simulink model "top12x17"  (Simulink 6.3)
settings: Solver=FixedStepDiscrete  StartTime=0.0  StopTime=5000  FixedStep=1  RelTol=1e-3
PreLoadFcn:
  | FifoDepth=17;
  | SymbolWidth = 8;
InitFcn:
  | %% DSPBuilder Start
  | alt_dspbuilder_update_model(bdroot)
  | %% DSPBuilder End
libraries: allblocks_alteradspbuilder2 x98, simulink x1
settings Model: LastModifiedBy=LKONG  StrictBusMsg=None
settings DataIOCC: SignalLoggingName=sigsOut
settings OptimizationCC: BooleanDataType=off  InlineInvariantSignals=on
settings DebuggingCC: SolverPrmCheckMsg=none
settings HardwareCC: TargetUnknown=on

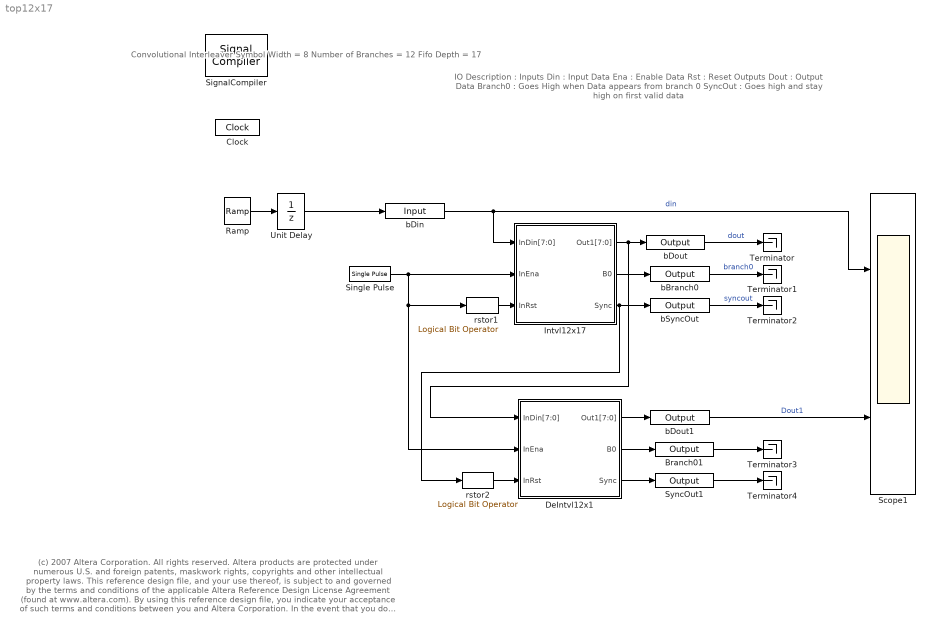
== system top12x17 ==
  note: (c) 2007 Altera Corporation. All rights reserved.  Altera products are protected under numerous U.S. and foreign patents, maskwork rights, copyrights and other intellectual property laws.
      | This reference design file, and your use thereof, is subject to and governed by the terms and conditions of the applicable Altera Reference Design License Agreement (found at www.altera.com).
      | By using this reference design file, you indicate your acceptance of such terms and conditions between you and Altera Corporation.
      | In the event that you do not agree with such terms and conditions, you may not use the reference design file and please promptly destroy any copies you have made.
      | This reference design file being provided on an "as-is" basis and as an accommodation and therefore all warranties, representations or guarantees of any kind (whether express, implied or statutory)
      | including, without limitation, warranties of merchantability, non-infringement, or fitness for a particular purpose, are specifically disclaimed.
      | By making this reference design file available, Altera expressly does not recommend, suggest or require that this reference design file be used in combination with any other product not provided by Altera
  note: IO Description :
      |
      | Inputs
      |            Din    : Input Data
      |            Ena   : Enable Data
      |            Rst    : Reset
      |
      | Outputs
      |           Dout        : Output Data
      |           Branch0 : Goes High when Data appears from branch 0
      |           SyncOut : Goes high and stay high on first valid data
  note: Convolutional Interleaver
      | Symbol Width = 8
      | Number of Branches = 12
      | Fifo Depth = 17
  Branch01 : allblocks_alteradspbuilder2/Output  iofile=d:\wsTrunk\workspace\Documentation\DesignExamples\Demos\Transforms\CrossInterleaver12x17\tb_top12x17\top12x17_Branch01.capture  BusType=Single Bit  bwl=1  bwr=0  PORTTYPE=Output
  Clock : allblocks_alteradspbuilder2/Clock  ClockPeriod=100  ClockPeriodUnit=ns  SampleTime=1  SimulationStartCycle=5  PhaseOffset=0  Reset=aclr  ResetType=Active Low  Export=off
  DeIntvl12x1 : Subsystem  AncestorBlock=ALTELINK/AltLab/HDL SubSystem
      mask Type: SubSystem AlteraBlockSet
  Intvl12x17 : Subsystem  AncestorBlock=ALTELINK/AltLab/HDL SubSystem
      mask Type: SubSystem AlteraBlockSet
  Ramp : simulink/Sources/Ramp  slope=1  start=0  X0=3
  Scope1 : Scope  NumInputPorts=2
      settings: TimeRange=3000  YMin=-5~-150  YMax=5~150
  SignalCompiler : allblocks_alteradspbuilder2/Signal Compiler  DeviceFamily=Cyclone IV GX  DeviceName=AUTO  EnableSignalTap=off  SignalTapDepth=128  UseBoardBlock=off  StpUseDefaultClock=on  StpClock=Clock
  Single Pulse : allblocks_alteradspbuilder2/Single Pulse  signal_type=Step Up  impulse_width=1  delay=1  SpecifyClock=off  use_ena=off  use_sclr=off
  SyncOut1 : allblocks_alteradspbuilder2/Output  iofile=d:\wsTrunk\workspace\Documentation\DesignExamples\Demos\Transforms\CrossInterleaver12x17\tb_top12x17\top12x17_SyncOut1.capture  BusType=Single Bit  bwl=1  bwr=0  PORTTYPE=Output
  Terminator{,1..4} (5 alike) : Terminator
  Unit Delay : UnitDelay
  bBranch0 : allblocks_alteradspbuilder2/Output  iofile=d:\wsTrunk\workspace\Documentation\DesignExamples\Demos\Transforms\CrossInterleaver12x17\tb_top12x17\top12x17_bBranch0.capture  BusType=Single Bit  bwl=1  bwr=0  PORTTYPE=Output
  bDin : allblocks_alteradspbuilder2/Input  iofile=d:\wsTrunk\workspace\Documentation\DesignExamples\Demos\Transforms\CrossInterleaver12x17\tb_top12x17\top12x17_bDin.salt  BusType=Signed Integer  bwl=8  bwr=0  SpecifyClock=off  PORTTYPE=Input
  bDout : allblocks_alteradspbuilder2/Output  iofile=d:\wsTrunk\workspace\Documentation\DesignExamples\Demos\Transforms\CrossInterleaver12x17\tb_top12x17\top12x17_bDout.capture  BusType=Signed Integer  bwl=8  bwr=0  PORTTYPE=Output
  bDout1 : allblocks_alteradspbuilder2/Output  iofile=d:\wsTrunk\workspace\Documentation\DesignExamples\Demos\Transforms\CrossInterleaver12x17\tb_top12x17\top12x17_bDout1.capture  BusType=Signed Integer  bwl=8  bwr=0  PORTTYPE=Output
  bSyncOut : allblocks_alteradspbuilder2/Output  iofile=d:\wsTrunk\workspace\Documentation\DesignExamples\Demos\Transforms\CrossInterleaver12x17\tb_top12x17\top12x17_bSyncOut.capture  BusType=Single Bit  bwl=1  bwr=0  PORTTYPE=Output
  rstor1 : allblocks_alteradspbuilder2/Logical Bit Operator  LogicalOperator=NOT  user_inputs=2
  rstor2 : allblocks_alteradspbuilder2/Logical Bit Operator  LogicalOperator=NOT  user_inputs=2
  wires:
  Intvl12x17/1(Out1[7:0]) -> bDout/1, DeIntvl12x1/1(InDin[7:0])
  bDin/1 -> Scope1/1, Intvl12x17/1(InDin[7:0])  "din"
  Single Pulse/1 -> Intvl12x17/2(InEna), rstor1/1, DeIntvl12x1/2(InEna)
  rstor1/1 -> Intvl12x17/3(InRst)
  Ramp/1 -> Unit Delay/1
  Intvl12x17/2(B0) -> bBranch0/1
  Intvl12x17/3(Sync) -> bSyncOut/1, rstor2/1
  Unit Delay/1 -> bDin/1
  rstor2/1 -> DeIntvl12x1/3(InRst)
  DeIntvl12x1/1(Out1[7:0]) -> bDout1/1
  DeIntvl12x1/2(B0) -> Branch01/1
  DeIntvl12x1/3(Sync) -> SyncOut1/1
  bDout/1 -> Terminator/1  "dout"
  bBranch0/1 -> Terminator1/1  "branch0"
  bSyncOut/1 -> Terminator2/1  "syncout"
  Branch01/1 -> Terminator3/1
  SyncOut1/1 -> Terminator4/1
  bDout1/1 -> Scope1/2  "Dout1"

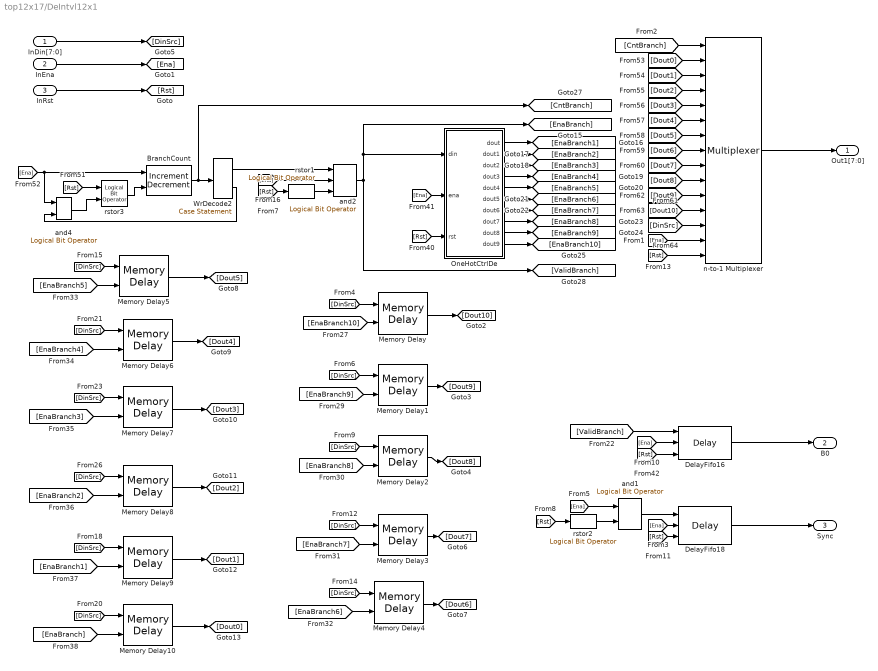
== system top12x17/DeIntvl12x1 ==
  InDin[7:0] : Inport
  InEna : Inport  Port=2
  InRst : Inport  Port=3
  BranchCount : allblocks_alteradspbuilder2/Increment Decrement  BusType=Unsigned Integer  bwl=4  bwr=0  SpecifyClock=off  clr_value=0  direction=Increment  phase_selection=1  use_ena=on  use_sclr=on
  DelayFifo16 : allblocks_alteradspbuilder2/Delay  pipeline=2  ClockPhase=1  use_ena=on  use_sclr=on  use_init=off  reset_value=1
  DelayFifo18 : allblocks_alteradspbuilder2/Delay  pipeline=2  ClockPhase=1  use_ena=on  use_sclr=on  use_init=off  reset_value=1
  Memory Delay : allblocks_alteradspbuilder2/Memory Delay  BusType=Inferred  bwl=8  bwr=0  pipeline=17  ram_type=AUTO  use_ena=on  use_sclr=off
  Memory Delay1 : allblocks_alteradspbuilder2/Memory Delay  BusType=Inferred  bwl=8  bwr=0  pipeline=34  ram_type=AUTO  use_ena=on  use_sclr=off
  Memory Delay10 : allblocks_alteradspbuilder2/Memory Delay  BusType=Inferred  bwl=8  bwr=0  pipeline=187  ram_type=AUTO  use_ena=on  use_sclr=off
  Memory Delay2 : allblocks_alteradspbuilder2/Memory Delay  BusType=Inferred  bwl=8  bwr=0  pipeline=51  ram_type=AUTO  use_ena=on  use_sclr=off
  Memory Delay3 : allblocks_alteradspbuilder2/Memory Delay  BusType=Inferred  bwl=8  bwr=0  pipeline=68  ram_type=AUTO  use_ena=on  use_sclr=off
  Memory Delay4 : allblocks_alteradspbuilder2/Memory Delay  BusType=Inferred  bwl=8  bwr=0  pipeline=85  ram_type=AUTO  use_ena=on  use_sclr=off
  Memory Delay5 : allblocks_alteradspbuilder2/Memory Delay  BusType=Inferred  bwl=8  bwr=0  pipeline=102  ram_type=AUTO  use_ena=on  use_sclr=off
  Memory Delay6 : allblocks_alteradspbuilder2/Memory Delay  BusType=Inferred  bwl=8  bwr=0  pipeline=119  ram_type=AUTO  use_ena=on  use_sclr=off
  Memory Delay7 : allblocks_alteradspbuilder2/Memory Delay  BusType=Inferred  bwl=8  bwr=0  pipeline=136  ram_type=AUTO  use_ena=on  use_sclr=off
  Memory Delay8 : allblocks_alteradspbuilder2/Memory Delay  BusType=Inferred  bwl=8  bwr=0  pipeline=153  ram_type=AUTO  use_ena=on  use_sclr=off
  Memory Delay9 : allblocks_alteradspbuilder2/Memory Delay  BusType=Inferred  bwl=8  bwr=0  pipeline=170  ram_type=AUTO  use_ena=on  use_sclr=off
  OneHotCtrlDe : Subsystem  AncestorBlock=ALTELINK/AltLab/HDL SubSystem
      mask Type: SubSystem AlteraBlockSet
  WrDecode2 : allblocks_alteradspbuilder2/Case Statement  numOutputs=2  case_expression=0,11  formatted_case_expression=00000000,00001011  BusType=Signed Integer  bwl=8  bwr=0  pipeline=off  hasDefault=off
  and1 : allblocks_alteradspbuilder2/Logical Bit Operator  LogicalOperator=AND  user_inputs=2
  and2 : allblocks_alteradspbuilder2/Logical Bit Operator  LogicalOperator=AND  user_inputs=3
  and4 : allblocks_alteradspbuilder2/Logical Bit Operator  LogicalOperator=AND  user_inputs=2
  n-to-1 Multiplexer : allblocks_alteradspbuilder2/Multiplexer  numInputs=12  pipeline=2  oneHot=off  use_ena=on  use_aclr=on
  rstor1 : allblocks_alteradspbuilder2/Logical Bit Operator  LogicalOperator=NOT  user_inputs=2
  rstor2 : allblocks_alteradspbuilder2/Logical Bit Operator  LogicalOperator=NOT  user_inputs=2
  rstor3 : allblocks_alteradspbuilder2/Logical Bit Operator  LogicalOperator=OR  user_inputs=2
  Out1[7:0] : Outport
  B0 : Outport  Port=2
  Sync : Outport  Port=3
  wires:
  and1/1 -> DelayFifo18/1
  rstor2/1 -> and1/2
  [Ena] -> and1/1
  [Rst] -> rstor2/1
  DelayFifo18/1 -> Sync/1
  [CntBranch] -> n-to-1 Multiplexer/1
  DelayFifo16/1 -> B0/1
  [ValidBranch] -> DelayFifo16/1
  [Rst] -> rstor1/1
  and2/1 -> [ValidBranch], OneHotCtrlDe/1(din), [EnaBranch]
  [DinSrc] -> n-to-1 Multiplexer/13
  [Dout10] -> n-to-1 Multiplexer/12
  [Dout9] -> n-to-1 Multiplexer/11
  [Dout8] -> n-to-1 Multiplexer/10
  [Dout7] -> n-to-1 Multiplexer/9
  [Dout6] -> n-to-1 Multiplexer/8
  [Dout5] -> n-to-1 Multiplexer/7
  [Dout4] -> n-to-1 Multiplexer/6
  [Dout3] -> n-to-1 Multiplexer/5
  [Dout2] -> n-to-1 Multiplexer/4
  [Dout1] -> n-to-1 Multiplexer/3
  [Dout0] -> n-to-1 Multiplexer/2
  [Ena] -> BranchCount/1, and4/1
  [Rst] -> rstor3/1
  rstor3/1 -> BranchCount/2
  BranchCount/1 -> WrDecode2/1, [CntBranch]
  [EnaBranch4] -> Memory Delay6/2
  [EnaBranch3] -> Memory Delay7/2
  [EnaBranch2] -> Memory Delay8/2
  [EnaBranch1] -> Memory Delay9/2
  [EnaBranch] -> Memory Delay10/2
  [EnaBranch5] -> Memory Delay5/2
  [EnaBranch6] -> Memory Delay4/2
  [EnaBranch7] -> Memory Delay3/2
  [EnaBranch8] -> Memory Delay2/2
  [EnaBranch9] -> Memory Delay1/2
  [EnaBranch10] -> Memory Delay/2
  Memory Delay10/1 -> [Dout0]
  Memory Delay9/1 -> [Dout1]
  Memory Delay8/1 -> [Dout2]
  Memory Delay7/1 -> [Dout3]
  Memory Delay6/1 -> [Dout4]
  Memory Delay5/1 -> [Dout5]
  Memory Delay4/1 -> [Dout6]
  Memory Delay3/1 -> [Dout7]
  Memory Delay2/1 -> [Dout8]
  Memory Delay1/1 -> [Dout9]
  Memory Delay/1 -> [Dout10]
  [DinSrc] -> Memory Delay10/1
  [DinSrc] -> Memory Delay9/1
  [DinSrc] -> Memory Delay8/1
  [DinSrc] -> Memory Delay7/1
  [DinSrc] -> Memory Delay6/1
  [DinSrc] -> Memory Delay5/1
  [DinSrc] -> Memory Delay4/1
  [DinSrc] -> Memory Delay3/1
  [DinSrc] -> Memory Delay2/1
  [DinSrc] -> Memory Delay1/1
  [DinSrc] -> Memory Delay/1
  InRst/1 -> [Rst]
  InEna/1 -> [Ena]
  InDin[7:0]/1 -> [DinSrc]
  n-to-1 Multiplexer/1 -> Out1[7:0]/1
  [Rst] -> DelayFifo16/3
  [Ena] -> DelayFifo16/2
  [Rst] -> OneHotCtrlDe/3(rst)
  [Ena] -> OneHotCtrlDe/2(ena)
  [Ena] -> n-to-1 Multiplexer/14
  [Rst] -> n-to-1 Multiplexer/15
  OneHotCtrlDe/1(dout) -> [EnaBranch1]
  OneHotCtrlDe/2(dout1) -> [EnaBranch2]
  OneHotCtrlDe/3(dout2) -> [EnaBranch3]
  OneHotCtrlDe/4(dout3) -> [EnaBranch4]
  OneHotCtrlDe/5(dout4) -> [EnaBranch5]
  OneHotCtrlDe/6(dout5) -> [EnaBranch6]
  OneHotCtrlDe/7(dout6) -> [EnaBranch7]
  OneHotCtrlDe/8(dout7) -> [EnaBranch8]
  OneHotCtrlDe/9(dout8) -> [EnaBranch9]
  OneHotCtrlDe/10(dout9) -> [EnaBranch10]
  [Rst] -> DelayFifo18/3
  [Ena] -> DelayFifo18/2
  [Ena] -> and2/2
  and4/1 -> rstor3/2
  WrDecode2/2 -> and4/2
  WrDecode2/1 -> and2/1
  rstor1/1 -> and2/3

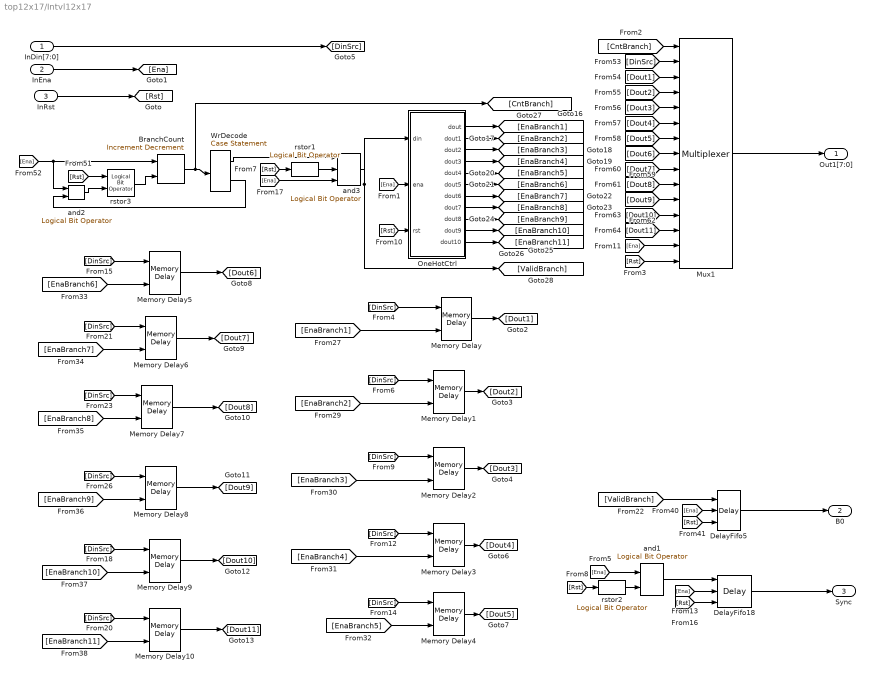
== system top12x17/Intvl12x17 ==
  InDin[7:0] : Inport
  InEna : Inport  Port=2
  InRst : Inport  Port=3
  BranchCount : allblocks_alteradspbuilder2/Increment Decrement  BusType=Unsigned Integer  bwl=4  bwr=0  SpecifyClock=off  clr_value=0  direction=Increment  phase_selection=1  use_ena=on  use_sclr=on
  DelayFifo18 : allblocks_alteradspbuilder2/Delay  pipeline=2  ClockPhase=1  use_ena=on  use_sclr=on  use_init=off  reset_value=1
  DelayFifo5 : allblocks_alteradspbuilder2/Delay  pipeline=2  ClockPhase=1  use_ena=on  use_sclr=on  use_init=off  reset_value=1
  Memory Delay : allblocks_alteradspbuilder2/Memory Delay  BusType=Inferred  bwl=8  bwr=0  pipeline=17  ram_type=AUTO  use_ena=on  use_sclr=off
  Memory Delay1 : allblocks_alteradspbuilder2/Memory Delay  BusType=Inferred  bwl=8  bwr=0  pipeline=34  ram_type=AUTO  use_ena=on  use_sclr=off
  Memory Delay10 : allblocks_alteradspbuilder2/Memory Delay  BusType=Inferred  bwl=8  bwr=0  pipeline=187  ram_type=AUTO  use_ena=on  use_sclr=off
  Memory Delay2 : allblocks_alteradspbuilder2/Memory Delay  BusType=Inferred  bwl=8  bwr=0  pipeline=51  ram_type=AUTO  use_ena=on  use_sclr=off
  Memory Delay3 : allblocks_alteradspbuilder2/Memory Delay  BusType=Inferred  bwl=8  bwr=0  pipeline=68  ram_type=AUTO  use_ena=on  use_sclr=off
  Memory Delay4 : allblocks_alteradspbuilder2/Memory Delay  BusType=Inferred  bwl=8  bwr=0  pipeline=85  ram_type=AUTO  use_ena=on  use_sclr=off
  Memory Delay5 : allblocks_alteradspbuilder2/Memory Delay  BusType=Inferred  bwl=8  bwr=0  pipeline=102  ram_type=AUTO  use_ena=on  use_sclr=off
  Memory Delay6 : allblocks_alteradspbuilder2/Memory Delay  BusType=Inferred  bwl=8  bwr=0  pipeline=119  ram_type=AUTO  use_ena=on  use_sclr=off
  Memory Delay7 : allblocks_alteradspbuilder2/Memory Delay  BusType=Inferred  bwl=8  bwr=0  pipeline=136  ram_type=AUTO  use_ena=on  use_sclr=off
  Memory Delay8 : allblocks_alteradspbuilder2/Memory Delay  BusType=Inferred  bwl=8  bwr=0  pipeline=153  ram_type=AUTO  use_ena=on  use_sclr=off
  Memory Delay9 : allblocks_alteradspbuilder2/Memory Delay  BusType=Inferred  bwl=8  bwr=0  pipeline=170  ram_type=AUTO  use_ena=on  use_sclr=off
  Mux1 : allblocks_alteradspbuilder2/Multiplexer  numInputs=12  pipeline=2  oneHot=off  use_ena=on  use_aclr=on
  OneHotCtrl : Subsystem  AncestorBlock=ALTELINK/AltLab/HDL SubSystem
      mask Type: SubSystem AlteraBlockSet
  WrDecode : allblocks_alteradspbuilder2/Case Statement  numOutputs=2  case_expression=0,11  formatted_case_expression=00000000,00001011  BusType=Signed Integer  bwl=8  bwr=0  pipeline=off  hasDefault=off
  and1 : allblocks_alteradspbuilder2/Logical Bit Operator  LogicalOperator=AND  user_inputs=2
  and2 : allblocks_alteradspbuilder2/Logical Bit Operator  LogicalOperator=AND  user_inputs=2
  and3 : allblocks_alteradspbuilder2/Logical Bit Operator  LogicalOperator=AND  user_inputs=3
  rstor1 : allblocks_alteradspbuilder2/Logical Bit Operator  LogicalOperator=NOT  user_inputs=2
  rstor2 : allblocks_alteradspbuilder2/Logical Bit Operator  LogicalOperator=NOT  user_inputs=2
  rstor3 : allblocks_alteradspbuilder2/Logical Bit Operator  LogicalOperator=OR  user_inputs=2
  Out1[7:0] : Outport
  B0 : Outport  Port=2
  Sync : Outport  Port=3
  wires:
  rstor2/1 -> and1/2
  [Ena] -> and1/1
  [Rst] -> rstor2/1
  DelayFifo18/1 -> Sync/1
  [CntBranch] -> Mux1/1
  DelayFifo5/1 -> B0/1
  [ValidBranch] -> DelayFifo5/1
  rstor1/1 -> and3/2
  [Rst] -> rstor1/1
  and3/1 -> [ValidBranch], OneHotCtrl/1(din)
  WrDecode/1 -> and3/1
  [Ena] -> BranchCount/1, and2/1
  [Rst] -> rstor3/1
  rstor3/1 -> BranchCount/2
  BranchCount/1 -> [CntBranch], WrDecode/1
  Mux1/1 -> Out1[7:0]/1
  [EnaBranch7] -> Memory Delay6/2
  [EnaBranch8] -> Memory Delay7/2
  [EnaBranch9] -> Memory Delay8/2
  [EnaBranch10] -> Memory Delay9/2
  [EnaBranch11] -> Memory Delay10/2
  [EnaBranch6] -> Memory Delay5/2
  [EnaBranch5] -> Memory Delay4/2
  [EnaBranch4] -> Memory Delay3/2
  [EnaBranch3] -> Memory Delay2/2
  [EnaBranch2] -> Memory Delay1/2
  Memory Delay10/1 -> [Dout11]
  Memory Delay9/1 -> [Dout10]
  Memory Delay8/1 -> [Dout9]
  Memory Delay7/1 -> [Dout8]
  Memory Delay6/1 -> [Dout7]
  Memory Delay5/1 -> [Dout6]
  Memory Delay4/1 -> [Dout5]
  Memory Delay3/1 -> [Dout4]
  Memory Delay2/1 -> [Dout3]
  Memory Delay1/1 -> [Dout2]
  Memory Delay/1 -> [Dout1]
  [DinSrc] -> Memory Delay10/1
  [DinSrc] -> Memory Delay9/1
  [DinSrc] -> Memory Delay8/1
  [DinSrc] -> Memory Delay7/1
  [DinSrc] -> Memory Delay6/1
  [DinSrc] -> Memory Delay5/1
  [DinSrc] -> Memory Delay4/1
  [DinSrc] -> Memory Delay3/1
  [DinSrc] -> Memory Delay2/1
  [DinSrc] -> Memory Delay1/1
  [DinSrc] -> Memory Delay/1
  InRst/1 -> [Rst]
  InEna/1 -> [Ena]
  InDin[7:0]/1 -> [DinSrc]
  [Ena] -> OneHotCtrl/2(ena)
  OneHotCtrl/1(dout) -> [EnaBranch1]
  OneHotCtrl/2(dout1) -> [EnaBranch2]
  OneHotCtrl/3(dout2) -> [EnaBranch3]
  OneHotCtrl/4(dout3) -> [EnaBranch4]
  OneHotCtrl/5(dout4) -> [EnaBranch5]
  OneHotCtrl/6(dout5) -> [EnaBranch6]
  OneHotCtrl/7(dout6) -> [EnaBranch7]
  OneHotCtrl/8(dout7) -> [EnaBranch8]
  OneHotCtrl/9(dout8) -> [EnaBranch9]
  OneHotCtrl/10(dout9) -> [EnaBranch10]
  OneHotCtrl/11(dout10) -> [EnaBranch11]
  [Rst] -> Mux1/15
  [Ena] -> Mux1/14
  [Rst] -> DelayFifo5/3
  [Ena] -> DelayFifo5/2
  [DinSrc] -> Mux1/2
  [Dout1] -> Mux1/3
  [Dout2] -> Mux1/4
  [Dout3] -> Mux1/5
  [Dout4] -> Mux1/6
  [Dout5] -> Mux1/7
  [Dout6] -> Mux1/8
  [Dout7] -> Mux1/9
  [Dout8] -> Mux1/10
  [Dout9] -> Mux1/11
  [Dout10] -> Mux1/12
  [Dout11] -> Mux1/13
  [Rst] -> OneHotCtrl/3(rst)
  [Ena] -> DelayFifo18/2
  [Rst] -> DelayFifo18/3
  [Ena] -> and3/3
  and1/1 -> DelayFifo18/1
  [EnaBranch1] -> Memory Delay/2
  and2/1 -> rstor3/2
  WrDecode/2 -> and2/2

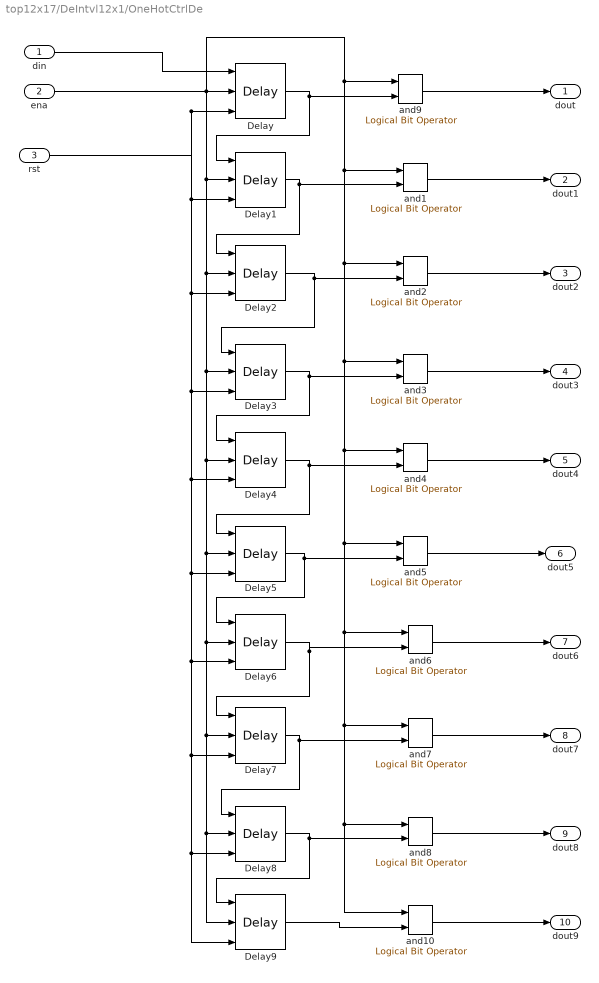
== system top12x17/DeIntvl12x1/OneHotCtrlDe ==
  din : Inport
  ena : Inport  Port=2
  rst : Inport  Port=3
  Delay{,1..9} (10 alike) : allblocks_alteradspbuilder2/Delay  pipeline=1  ClockPhase=1  use_ena=on  use_sclr=on  use_init=off  reset_value=1
  and{1..10} (10 alike) : allblocks_alteradspbuilder2/Logical Bit Operator  LogicalOperator=AND  user_inputs=2
  dout : Outport
  dout1 : Outport  Port=2
  dout2 : Outport  Port=3
  dout3 : Outport  Port=4
  dout4 : Outport  Port=5
  dout5 : Outport  Port=6
  dout6 : Outport  Port=7
  dout7 : Outport  Port=8
  dout8 : Outport  Port=9
  dout9 : Outport  Port=10
  wires:
  ena/1 -> Delay/2, Delay1/2, Delay2/2, Delay3/2, Delay4/2, Delay5/2, Delay8/2, Delay9/2, Delay7/2, Delay6/2, and9/1, and1/1, and10/1, and8/1, and7/1, and6/1, and5/1, and4/1, and3/1, and2/1
  din/1 -> Delay/1
  rst/1 -> Delay/3, Delay1/3, Delay2/3, Delay4/3, Delay5/3, Delay7/3, Delay8/3, Delay9/3, Delay6/3, Delay3/3
  Delay1/1 -> Delay2/1, and1/2
  Delay2/1 -> Delay3/1, and2/2
  Delay3/1 -> Delay4/1, and3/2
  Delay4/1 -> Delay5/1, and4/2
  Delay5/1 -> Delay6/1, and5/2
  Delay6/1 -> Delay7/1, and6/2
  Delay7/1 -> Delay8/1, and7/2
  Delay8/1 -> Delay9/1, and8/2
  Delay/1 -> Delay1/1, and9/2
  and9/1 -> dout/1
  and1/1 -> dout1/1
  and2/1 -> dout2/1
  and3/1 -> dout3/1
  and4/1 -> dout4/1
  and5/1 -> dout5/1
  and6/1 -> dout6/1
  and7/1 -> dout7/1
  and8/1 -> dout8/1
  and10/1 -> dout9/1
  Delay9/1 -> and10/2

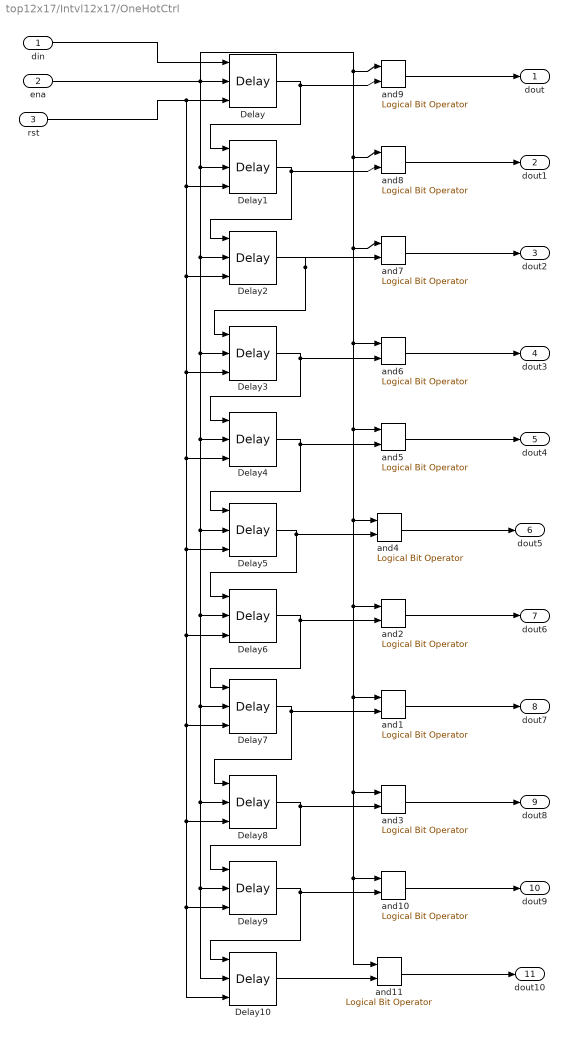
== system top12x17/Intvl12x17/OneHotCtrl ==
  din : Inport
  ena : Inport  Port=2
  rst : Inport  Port=3
  Delay{,1..10} (11 alike) : allblocks_alteradspbuilder2/Delay  pipeline=1  ClockPhase=1  use_ena=on  use_sclr=on  use_init=off  reset_value=1
  and{1..11} (11 alike) : allblocks_alteradspbuilder2/Logical Bit Operator  LogicalOperator=AND  user_inputs=2
  dout : Outport
  dout1 : Outport  Port=2
  dout2 : Outport  Port=3
  dout3 : Outport  Port=4
  dout4 : Outport  Port=5
  dout5 : Outport  Port=6
  dout6 : Outport  Port=7
  dout7 : Outport  Port=8
  dout8 : Outport  Port=9
  dout9 : Outport  Port=10
  dout10 : Outport  Port=11
  wires:
  ena/1 -> Delay/2, Delay1/2, Delay2/2, Delay3/2, Delay4/2, Delay5/2, Delay8/2, Delay9/2, Delay10/2, Delay7/2, Delay6/2, and9/1, and8/1, and7/1, and6/1, and5/1, and4/1, and2/1, and1/1, and3/1, and11/1, and10/1
  din/1 -> Delay/1
  rst/1 -> Delay/3, Delay1/3, Delay2/3, Delay4/3, Delay5/3, Delay7/3, Delay10/3, Delay9/3, Delay8/3, Delay6/3, Delay3/3
  Delay1/1 -> Delay2/1, and8/2
  Delay2/1 -> Delay3/1, and7/2
  Delay3/1 -> Delay4/1, and6/2
  Delay4/1 -> Delay5/1, and5/2
  Delay5/1 -> Delay6/1, and4/2
  Delay6/1 -> Delay7/1, and2/2
  Delay7/1 -> Delay8/1, and1/2
  Delay8/1 -> Delay9/1, and3/2
  Delay9/1 -> Delay10/1, and10/2
  Delay/1 -> Delay1/1, and9/2
  and3/1 -> dout8/1
  and1/1 -> dout7/1
  and2/1 -> dout6/1
  and4/1 -> dout5/1
  and5/1 -> dout4/1
  and7/1 -> dout2/1
  and8/1 -> dout1/1
  and9/1 -> dout/1
  and10/1 -> dout9/1
  and11/1 -> dout10/1
  Delay10/1 -> and11/2
  and6/1 -> dout3/1
